simulink model "ass"  (Simulink 6.5)
settings: Solver=ode45  StartTime=0.0  StopTime=10.0  RelTol=1e-3
libraries: cdsFilt x333, cdsPhase x144, cdsRfmIO x26, cdsOsc x18, cdsMuxMatrix x8, cdsEpicsOut x3, cdsEzCaRead x1, cdsEpicsIn x1, cdsBitwise x1, cdsParameters x1
(part 3 of 17)

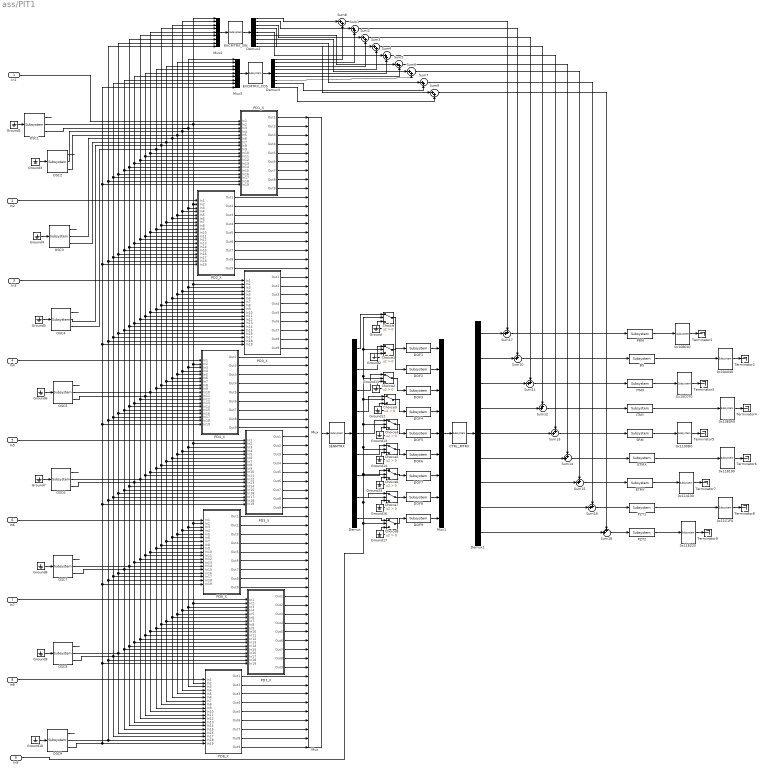
== system ass/PIT1 ==
  In1 : Inport
  In2 : Inport  Port=2
  In3 : Inport  Port=3
  In4 : Inport  Port=4
  In5 : Inport  Port=5
  In6 : Inport  Port=6
  In7 : Inport  Port=7
  In8 : Inport  Port=8
  In9 : Inport  Port=9
  0x108010 : cdsRfmIO/Subsystem  Tag=cdsRfmIO  Description=VMIC5565 Reflective Memory read/write  SystemSampleTime=-1
      settings: AttributesFormatString=%<Tag>
  0x10A040 : cdsRfmIO/Subsystem  Tag=cdsRfmIO  Description=VMIC5565 Reflective Memory read/write  SystemSampleTime=-1
      settings: AttributesFormatString=%<Tag>
  0x10C070 : cdsRfmIO/Subsystem  Tag=cdsRfmIO  Description=VMIC5565 Reflective Memory read/write  SystemSampleTime=-1
      settings: AttributesFormatString=%<Tag>
  0x10E0A0 : cdsRfmIO/Subsystem  Tag=cdsRfmIO  Description=VMIC5565 Reflective Memory read/write  SystemSampleTime=-1
      settings: AttributesFormatString=%<Tag>
  0x1100D0 : cdsRfmIO/Subsystem  Tag=cdsRfmIO  Description=VMIC5565 Reflective Memory read/write  SystemSampleTime=-1
      settings: AttributesFormatString=%<Tag>
  0x114130 : cdsRfmIO/Subsystem  Tag=cdsRfmIO  Description=VMIC5565 Reflective Memory read/write  SystemSampleTime=-1
      settings: AttributesFormatString=%<Tag>
  0x118190 : cdsRfmIO/Subsystem  Tag=cdsRfmIO  Description=VMIC5565 Reflective Memory read/write  SystemSampleTime=-1
      settings: AttributesFormatString=%<Tag>
  0x11C1F0 : cdsRfmIO/Subsystem  Tag=cdsRfmIO  Description=VMIC5565 Reflective Memory read/write  SystemSampleTime=-1
      settings: AttributesFormatString=%<Tag>
  0x11E220 : cdsRfmIO/Subsystem  Tag=cdsRfmIO  Description=VMIC5565 Reflective Memory read/write  SystemSampleTime=-1
      settings: AttributesFormatString=%<Tag>
  BS : cdsFilt/Subsystem  Tag=cdsFilt  Description=|  SystemSampleTime=-1
      | Purpose:                                                                                                                                                                                                                                  
      | Standard CDS IIR filter module.                                                                                                                                                                                                           
      |                                                                                                                                                                                                                                           
      | Operation:                                                                                                                                                                                                                                
      | Consists of 10 second order section IIR filters, plus a ramped gain stage. In FE code, also provides pre-defined test points and excitation channel inputs. The filter coefficients are defined in the LIGO system using the 'foton' tool.
      |                                                                                                                                                                                                                                           
      | Usage:                                                                                                                                                                                                                                    
      | Name the part with the desired filter module name.
      settings: AttributesFormatString=%<Tag>
  CTRL_MTRX : cdsMuxMatrix/Subsystem  Tag=cdsMuxMatrix  Description=Any size matrix. Inputs and outputs must be connected using Mux and Demux parts.  SystemSampleTime=-1
      settings: AttributesFormatString=%<Tag>
  Choice{,1..8} (9 alike) : Switch  Criteria=u2 > Threshold
  DOF1 : cdsFilt/Subsystem  Tag=cdsFilt  Description=|  SystemSampleTime=-1
      | Purpose:                                                                                                                                                                                                                                  
      | Standard CDS IIR filter module.                                                                                                                                                                                                           
      |                                                                                                                                                                                                                                           
      | Operation:                                                                                                                                                                                                                                
      | Consists of 10 second order section IIR filters, plus a ramped gain stage. In FE code, also provides pre-defined test points and excitation channel inputs. The filter coefficients are defined in the LIGO system using the 'foton' tool.
      |                                                                                                                                                                                                                                           
      | Usage:                                                                                                                                                                                                                                    
      | Name the part with the desired filter module name.
      settings: AttributesFormatString=%<Tag>
  DOF2 : cdsFilt/Subsystem  Tag=cdsFilt  Description=|  SystemSampleTime=-1
      | Purpose:                                                                                                                                                                                                                                  
      | Standard CDS IIR filter module.                                                                                                                                                                                                           
      |                                                                                                                                                                                                                                           
      | Operation:                                                                                                                                                                                                                                
      | Consists of 10 second order section IIR filters, plus a ramped gain stage. In FE code, also provides pre-defined test points and excitation channel inputs. The filter coefficients are defined in the LIGO system using the 'foton' tool.
      |                                                                                                                                                                                                                                           
      | Usage:                                                                                                                                                                                                                                    
      | Name the part with the desired filter module name.
      settings: AttributesFormatString=%<Tag>
  DOF3 : cdsFilt/Subsystem  Tag=cdsFilt  Description=|  SystemSampleTime=-1
      | Purpose:                                                                                                                                                                                                                                  
      | Standard CDS IIR filter module.                                                                                                                                                                                                           
      |                                                                                                                                                                                                                                           
      | Operation:                                                                                                                                                                                                                                
      | Consists of 10 second order section IIR filters, plus a ramped gain stage. In FE code, also provides pre-defined test points and excitation channel inputs. The filter coefficients are defined in the LIGO system using the 'foton' tool.
      |                                                                                                                                                                                                                                           
      | Usage:                                                                                                                                                                                                                                    
      | Name the part with the desired filter module name.
      settings: AttributesFormatString=%<Tag>
  DOF4 : cdsFilt/Subsystem  Tag=cdsFilt  Description=|  SystemSampleTime=-1
      | Purpose:                                                                                                                                                                                                                                  
      | Standard CDS IIR filter module.                                                                                                                                                                                                           
      |                                                                                                                                                                                                                                           
      | Operation:                                                                                                                                                                                                                                
      | Consists of 10 second order section IIR filters, plus a ramped gain stage. In FE code, also provides pre-defined test points and excitation channel inputs. The filter coefficients are defined in the LIGO system using the 'foton' tool.
      |                                                                                                                                                                                                                                           
      | Usage:                                                                                                                                                                                                                                    
      | Name the part with the desired filter module name.
      settings: AttributesFormatString=%<Tag>
  DOF5 : cdsFilt/Subsystem  Tag=cdsFilt  Description=|  SystemSampleTime=-1
      | Purpose:                                                                                                                                                                                                                                  
      | Standard CDS IIR filter module.                                                                                                                                                                                                           
      |                                                                                                                                                                                                                                           
      | Operation:                                                                                                                                                                                                                                
      | Consists of 10 second order section IIR filters, plus a ramped gain stage. In FE code, also provides pre-defined test points and excitation channel inputs. The filter coefficients are defined in the LIGO system using the 'foton' tool.
      |                                                                                                                                                                                                                                           
      | Usage:                                                                                                                                                                                                                                    
      | Name the part with the desired filter module name.
      settings: AttributesFormatString=%<Tag>
  DOF6 : cdsFilt/Subsystem  Tag=cdsFilt  Description=|  SystemSampleTime=-1
      | Purpose:                                                                                                                                                                                                                                  
      | Standard CDS IIR filter module.                                                                                                                                                                                                           
      |                                                                                                                                                                                                                                           
      | Operation:                                                                                                                                                                                                                                
      | Consists of 10 second order section IIR filters, plus a ramped gain stage. In FE code, also provides pre-defined test points and excitation channel inputs. The filter coefficients are defined in the LIGO system using the 'foton' tool.
      |                                                                                                                                                                                                                                           
      | Usage:                                                                                                                                                                                                                                    
      | Name the part with the desired filter module name.
      settings: AttributesFormatString=%<Tag>
  DOF7 : cdsFilt/Subsystem  Tag=cdsFilt  Description=|  SystemSampleTime=-1
      | Purpose:                                                                                                                                                                                                                                  
      | Standard CDS IIR filter module.                                                                                                                                                                                                           
      |                                                                                                                                                                                                                                           
      | Operation:                                                                                                                                                                                                                                
      | Consists of 10 second order section IIR filters, plus a ramped gain stage. In FE code, also provides pre-defined test points and excitation channel inputs. The filter coefficients are defined in the LIGO system using the 'foton' tool.
      |                                                                                                                                                                                                                                           
      | Usage:                                                                                                                                                                                                                                    
      | Name the part with the desired filter module name.
      settings: AttributesFormatString=%<Tag>
  DOF8 : cdsFilt/Subsystem  Tag=cdsFilt  Description=|  SystemSampleTime=-1
      | Purpose:                                                                                                                                                                                                                                  
      | Standard CDS IIR filter module.                                                                                                                                                                                                           
      |                                                                                                                                                                                                                                           
      | Operation:                                                                                                                                                                                                                                
      | Consists of 10 second order section IIR filters, plus a ramped gain stage. In FE code, also provides pre-defined test points and excitation channel inputs. The filter coefficients are defined in the LIGO system using the 'foton' tool.
      |                                                                                                                                                                                                                                           
      | Usage:                                                                                                                                                                                                                                    
      | Name the part with the desired filter module name.
      settings: AttributesFormatString=%<Tag>
  DOF9 : cdsFilt/Subsystem  Tag=cdsFilt  Description=|  SystemSampleTime=-1
      | Purpose:                                                                                                                                                                                                                                  
      | Standard CDS IIR filter module.                                                                                                                                                                                                           
      |                                                                                                                                                                                                                                           
      | Operation:                                                                                                                                                                                                                                
      | Consists of 10 second order section IIR filters, plus a ramped gain stage. In FE code, also provides pre-defined test points and excitation channel inputs. The filter coefficients are defined in the LIGO system using the 'foton' tool.
      |                                                                                                                                                                                                                                           
      | Usage:                                                                                                                                                                                                                                    
      | Name the part with the desired filter module name.
      settings: AttributesFormatString=%<Tag>
  Demux{,1..3} (4 alike) : Demux  Outputs=9
  ETMX : cdsFilt/Subsystem  Tag=cdsFilt  Description=|  SystemSampleTime=-1
      | Purpose:                                                                                                                                                                                                                                  
      | Standard CDS IIR filter module.                                                                                                                                                                                                           
      |                                                                                                                                                                                                                                           
      | Operation:                                                                                                                                                                                                                                
      | Consists of 10 second order section IIR filters, plus a ramped gain stage. In FE code, also provides pre-defined test points and excitation channel inputs. The filter coefficients are defined in the LIGO system using the 'foton' tool.
      |                                                                                                                                                                                                                                           
      | Usage:                                                                                                                                                                                                                                    
      | Name the part with the desired filter module name.
      settings: AttributesFormatString=%<Tag>
  ETMY : cdsFilt/Subsystem  Tag=cdsFilt  Description=|  SystemSampleTime=-1
      | Purpose:                                                                                                                                                                                                                                  
      | Standard CDS IIR filter module.                                                                                                                                                                                                           
      |                                                                                                                                                                                                                                           
      | Operation:                                                                                                                                                                                                                                
      | Consists of 10 second order section IIR filters, plus a ramped gain stage. In FE code, also provides pre-defined test points and excitation channel inputs. The filter coefficients are defined in the LIGO system using the 'foton' tool.
      |                                                                                                                                                                                                                                           
      | Usage:                                                                                                                                                                                                                                    
      | Name the part with the desired filter module name.
      settings: AttributesFormatString=%<Tag>
  EXCMTRX_COS : cdsMuxMatrix/Subsystem  Tag=cdsMuxMatrix  Description=Any size matrix. Inputs and outputs must be connected using Mux and Demux parts.  SystemSampleTime=-1
      settings: AttributesFormatString=%<Tag>
  EXCMTRX_SIN : cdsMuxMatrix/Subsystem  Tag=cdsMuxMatrix  Description=Any size matrix. Inputs and outputs must be connected using Mux and Demux parts.  SystemSampleTime=-1
      settings: AttributesFormatString=%<Tag>
  Ground{,1..17} (18 alike) : Ground
  ITMX : cdsFilt/Subsystem  Tag=cdsFilt  Description=|  SystemSampleTime=-1
      | Purpose:                                                                                                                                                                                                                                  
      | Standard CDS IIR filter module.                                                                                                                                                                                                           
      |                                                                                                                                                                                                                                           
      | Operation:                                                                                                                                                                                                                                
      | Consists of 10 second order section IIR filters, plus a ramped gain stage. In FE code, also provides pre-defined test points and excitation channel inputs. The filter coefficients are defined in the LIGO system using the 'foton' tool.
      |                                                                                                                                                                                                                                           
      | Usage:                                                                                                                                                                                                                                    
      | Name the part with the desired filter module name.
      settings: AttributesFormatString=%<Tag>
  ITMY : cdsFilt/Subsystem  Tag=cdsFilt  Description=|  SystemSampleTime=-1
      | Purpose:                                                                                                                                                                                                                                  
      | Standard CDS IIR filter module.                                                                                                                                                                                                           
      |                                                                                                                                                                                                                                           
      | Operation:                                                                                                                                                                                                                                
      | Consists of 10 second order section IIR filters, plus a ramped gain stage. In FE code, also provides pre-defined test points and excitation channel inputs. The filter coefficients are defined in the LIGO system using the 'foton' tool.
      |                                                                                                                                                                                                                                           
      | Usage:                                                                                                                                                                                                                                    
      | Name the part with the desired filter module name.
      settings: AttributesFormatString=%<Tag>
  Mux : Mux  Inputs=72
  Mux1 : Mux  Inputs=9
  Mux2 : Mux  Inputs=9
  Mux3 : Mux  Inputs=9
  OSC{1..9} (9 alike) : cdsOsc/Subsystem  Tag=cdsOsc  Description=Oscillator  SystemSampleTime=-1
      settings: AttributesFormatString=%<Tag>
  PD1_X : Subsystem
  PD2_X : Subsystem
  PD3_X : Subsystem
  PD4_X : Subsystem
  PD5_X : Subsystem
  PD6_X : Subsystem
  PD7_X : Subsystem
  PD8_X : Subsystem
  PRM : cdsFilt/Subsystem  Tag=cdsFilt  Description=|  SystemSampleTime=-1
      | Purpose:                                                                                                                                                                                                                                  
      | Standard CDS IIR filter module.                                                                                                                                                                                                           
      |                                                                                                                                                                                                                                           
      | Operation:                                                                                                                                                                                                                                
      | Consists of 10 second order section IIR filters, plus a ramped gain stage. In FE code, also provides pre-defined test points and excitation channel inputs. The filter coefficients are defined in the LIGO system using the 'foton' tool.
      |                                                                                                                                                                                                                                           
      | Usage:                                                                                                                                                                                                                                    
      | Name the part with the desired filter module name.
      settings: AttributesFormatString=%<Tag>
  PZT1 : cdsFilt/Subsystem  Tag=cdsFilt  Description=|  SystemSampleTime=-1
      | Purpose:                                                                                                                                                                                                                                  
      | Standard CDS IIR filter module.                                                                                                                                                                                                           
      |                                                                                                                                                                                                                                           
      | Operation:                                                                                                                                                                                                                                
      | Consists of 10 second order section IIR filters, plus a ramped gain stage. In FE code, also provides pre-defined test points and excitation channel inputs. The filter coefficients are defined in the LIGO system using the 'foton' tool.
      |                                                                                                                                                                                                                                           
      | Usage:                                                                                                                                                                                                                                    
      | Name the part with the desired filter module name.
      settings: AttributesFormatString=%<Tag>
  PZT2 : cdsFilt/Subsystem  Tag=cdsFilt  Description=|  SystemSampleTime=-1
      | Purpose:                                                                                                                                                                                                                                  
      | Standard CDS IIR filter module.                                                                                                                                                                                                           
      |                                                                                                                                                                                                                                           
      | Operation:                                                                                                                                                                                                                                
      | Consists of 10 second order section IIR filters, plus a ramped gain stage. In FE code, also provides pre-defined test points and excitation channel inputs. The filter coefficients are defined in the LIGO system using the 'foton' tool.
      |                                                                                                                                                                                                                                           
      | Usage:                                                                                                                                                                                                                                    
      | Name the part with the desired filter module name.
      settings: AttributesFormatString=%<Tag>
  SENMTRX : cdsMuxMatrix/Subsystem  Tag=cdsMuxMatrix  Description=Any size matrix. Inputs and outputs must be connected using Mux and Demux parts.  SystemSampleTime=-1
      settings: AttributesFormatString=%<Tag>
  SRM : cdsFilt/Subsystem  Tag=cdsFilt  Description=|  SystemSampleTime=-1
      | Purpose:                                                                                                                                                                                                                                  
      | Standard CDS IIR filter module.                                                                                                                                                                                                           
      |                                                                                                                                                                                                                                           
      | Operation:                                                                                                                                                                                                                                
      | Consists of 10 second order section IIR filters, plus a ramped gain stage. In FE code, also provides pre-defined test points and excitation channel inputs. The filter coefficients are defined in the LIGO system using the 'foton' tool.
      |                                                                                                                                                                                                                                           
      | Usage:                                                                                                                                                                                                                                    
      | Name the part with the desired filter module name.
      settings: AttributesFormatString=%<Tag>
  Sum{1..9} (9 alike) : Sum  Inputs=|++
  Sum{10..18} (9 alike) : Sum  Inputs=++|
  Terminator{1..9} (9 alike) : Terminator
  wires:
  Ground1/1 -> OSC1/1
  PD1_X/1(Out1) -> Mux/1
  Mux/1 -> SENMTRX/1
  Mux1/1 -> CTRL_MTRX/1
  CTRL_MTRX/1 -> Demux1/1
  DOF1/1 -> Mux1/1
  DOF2/1 -> Mux1/2
  DOF3/1 -> Mux1/3
  DOF4/1 -> Mux1/4
  DOF5/1 -> Mux1/5
  DOF6/1 -> Mux1/6
  DOF7/1 -> Mux1/7
  DOF8/1 -> Mux1/8
  DOF9/1 -> Mux1/9
  0x108010/1 -> Terminator1/1
  0x10A040/1 -> Terminator2/1
  0x10C070/1 -> Terminator3/1
  0x10E0A0/1 -> Terminator4/1
  0x1100D0/1 -> Terminator5/1
  0x118190/1 -> Terminator6/1
  0x114130/1 -> Terminator7/1
  0x11C1F0/1 -> Terminator8/1
  0x11E220/1 -> Terminator9/1
  Ground3/1 -> OSC2/1
  Ground4/1 -> OSC3/1
  Ground5/1 -> OSC4/1
  Ground6/1 -> OSC5/1
  Ground7/1 -> OSC6/1
  Ground8/1 -> OSC7/1
  Ground9/1 -> OSC8/1
  Ground10/1 -> OSC9/1
  PD1_X/2(Out2) -> Mux/2
  PD1_X/3(Out3) -> Mux/3
  PD1_X/4(Out4) -> Mux/4
  PD1_X/5(Out5) -> Mux/5
  PD1_X/6(Out6) -> Mux/6
  PD1_X/7(Out7) -> Mux/7
  PD1_X/8(Out8) -> Mux/8
  PD1_X/9(Out9) -> Mux/9
  PD2_X/1(Out1) -> Mux/10
  PD2_X/2(Out2) -> Mux/11
  PD2_X/3(Out3) -> Mux/12
  PD2_X/4(Out4) -> Mux/13
  PD2_X/5(Out5) -> Mux/14
  PD2_X/6(Out6) -> Mux/15
  PD2_X/7(Out7) -> Mux/16
  PD2_X/8(Out8) -> Mux/17
  PD2_X/9(Out9) -> Mux/18
  PD3_X/1(Out1) -> Mux/19
  PD3_X/2(Out2) -> Mux/20
  PD3_X/3(Out3) -> Mux/21
  PD3_X/4(Out4) -> Mux/22
  PD3_X/5(Out5) -> Mux/23
  PD3_X/6(Out6) -> Mux/24
  PD3_X/7(Out7) -> Mux/25
  PD3_X/8(Out8) -> Mux/26
  PD3_X/9(Out9) -> Mux/27
  PD4_X/1(Out1) -> Mux/28
  PD4_X/2(Out2) -> Mux/29
  PD4_X/3(Out3) -> Mux/30
  PD4_X/4(Out4) -> Mux/31
  PD4_X/5(Out5) -> Mux/32
  PD4_X/6(Out6) -> Mux/33
  PD4_X/7(Out7) -> Mux/34
  PD4_X/8(Out8) -> Mux/35
  PD4_X/9(Out9) -> Mux/36
  PD5_X/1(Out1) -> Mux/37
  PD5_X/2(Out2) -> Mux/38
  PD5_X/3(Out3) -> Mux/39
  PD5_X/4(Out4) -> Mux/40
  PD5_X/5(Out5) -> Mux/41
  PD5_X/6(Out6) -> Mux/42
  PD5_X/7(Out7) -> Mux/43
  PD5_X/8(Out8) -> Mux/44
  PD5_X/9(Out9) -> Mux/45
  PD6_X/1(Out1) -> Mux/46
  PD6_X/2(Out2) -> Mux/47
  PD6_X/3(Out3) -> Mux/48
  PD6_X/4(Out4) -> Mux/49
  PD6_X/5(Out5) -> Mux/50
  PD6_X/6(Out6) -> Mux/51
  PD6_X/7(Out7) -> Mux/52
  PD6_X/8(Out8) -> Mux/53
  PD6_X/9(Out9) -> Mux/54
  PD7_X/1(Out1) -> Mux/55
  PD7_X/2(Out2) -> Mux/56
  PD7_X/3(Out3) -> Mux/57
  PD7_X/4(Out4) -> Mux/58
  PD7_X/5(Out5) -> Mux/59
  PD7_X/6(Out6) -> Mux/60
  PD7_X/7(Out7) -> Mux/61
  PD7_X/8(Out8) -> Mux/62
  PD7_X/9(Out9) -> Mux/63
  PD8_X/1(Out1) -> Mux/64
  PD8_X/2(Out2) -> Mux/65
  PD8_X/3(Out3) -> Mux/66
  PD8_X/4(Out4) -> Mux/67
  PD8_X/5(Out5) -> Mux/68
  PD8_X/6(Out6) -> Mux/69
  PD8_X/7(Out7) -> Mux/70
  PD8_X/8(Out8) -> Mux/71
  PD8_X/9(Out9) -> Mux/72
  OSC1/2 -> PD1_X/2(In2), PD7_X/2(In2), PD8_X/2(In2), PD6_X/2(In2), PD5_X/2(In2), PD4_X/2(In2), PD3_X/2(In2), PD2_X/2(In2), Mux2/1
  Mux2/1 -> EXCMTRX_SIN/1
  EXCMTRX_SIN/1 -> Demux2/1
  Mux3/1 -> EXCMTRX_COS/1
  EXCMTRX_COS/1 -> Demux3/1
  OSC1/3 -> PD7_X/3(In3), PD8_X/3(In3), PD6_X/3(In3), PD5_X/3(In3), PD4_X/3(In3), PD3_X/3(In3), PD2_X/3(In3), PD1_X/3(In3), Mux3/1
  OSC2/2 -> PD1_X/4(In4), Mux2/2, PD7_X/4(In4), PD8_X/4(In4), PD6_X/4(In4), PD5_X/4(In4), PD4_X/4(In4), PD3_X/4(In4), PD2_X/4(In4)
  OSC2/3 -> PD1_X/5(In5), Mux3/2, PD7_X/5(In5), PD8_X/5(In5), PD6_X/5(In5), PD5_X/5(In5), PD4_X/5(In5), PD3_X/5(In5), PD2_X/5(In5)
  OSC3/2 -> PD1_X/6(In6), Mux2/3, PD7_X/6(In6), PD8_X/6(In6), PD6_X/6(In6), PD5_X/6(In6), PD4_X/6(In6), PD3_X/6(In6), PD2_X/6(In6)
  OSC3/3 -> PD1_X/7(In7), Mux3/3, PD7_X/7(In7), PD8_X/7(In7), PD6_X/7(In7), PD5_X/7(In7), PD4_X/7(In7), PD3_X/7(In7), PD2_X/7(In7)
  OSC4/2 -> PD1_X/8(In8), PD7_X/8(In8), PD8_X/8(In8), PD6_X/8(In8), PD5_X/8(In8), PD4_X/8(In8), PD3_X/8(In8), PD2_X/8(In8), Mux2/4
  OSC4/3 -> PD1_X/9(In9), Mux3/4, PD7_X/9(In9), PD8_X/9(In9), PD6_X/9(In9), PD5_X/9(In9), PD4_X/9(In9), PD3_X/9(In9), PD2_X/9(In9)
  OSC5/2 -> PD1_X/10(In10), Mux2/5, PD2_X/10(In10), PD3_X/10(In10), PD7_X/10(In10), PD8_X/10(In10), PD6_X/10(In10), PD5_X/10(In10), PD4_X/10(In10)
  OSC5/3 -> PD1_X/11(In11), Mux3/5, PD2_X/11(In11), PD3_X/11(In11), PD7_X/11(In11), PD8_X/11(In11), PD6_X/11(In11), PD5_X/11(In11), PD4_X/11(In11)
  OSC6/2 -> PD1_X/12(In12), Mux2/6, PD2_X/12(In12), PD3_X/12(In12), PD4_X/12(In12), PD7_X/12(In12), PD8_X/12(In12), PD6_X/12(In12), PD5_X/12(In12)
  OSC6/3 -> PD1_X/13(In13), Mux3/6, PD2_X/13(In13), PD3_X/13(In13), PD4_X/13(In13), PD7_X/13(In13), PD8_X/13(In13), PD6_X/13(In13), PD5_X/13(In13)
  OSC7/2 -> PD1_X/14(In14), Mux2/7, PD2_X/14(In14), PD3_X/14(In14), PD4_X/14(In14), PD5_X/14(In14), PD7_X/14(In14), PD8_X/14(In14), PD6_X/14(In14)
  OSC7/3 -> PD1_X/15(In15), Mux3/7, PD2_X/15(In15), PD3_X/15(In15), PD4_X/15(In15), PD5_X/15(In15), PD7_X/15(In15), PD8_X/15(In15), PD6_X/15(In15)
  OSC8/2 -> PD1_X/16(In16), Mux2/8, PD2_X/16(In16), PD3_X/16(In16), PD4_X/16(In16), PD5_X/16(In16), PD6_X/16(In16), PD7_X/16(In16), PD8_X/16(In16)
  OSC8/3 -> PD1_X/17(In17), Mux3/8, PD2_X/17(In17), PD3_X/17(In17), PD4_X/17(In17), PD5_X/17(In17), PD6_X/17(In17), PD7_X/17(In17), PD8_X/17(In17)
  OSC9/2 -> PD1_X/18(In18), Mux2/9, PD2_X/18(In18), PD3_X/18(In18), PD4_X/18(In18), PD5_X/18(In18), PD6_X/18(In18), PD7_X/18(In18), PD8_X/18(In18)
  OSC9/3 -> PD1_X/19(In19), Mux3/9, PD2_X/19(In19), PD3_X/19(In19), PD4_X/19(In19), PD5_X/19(In19), PD6_X/19(In19), PD7_X/19(In19), PD8_X/19(In19)
  Demux2/1 -> Sum8/1
  Demux3/1 -> Sum8/2
  Demux2/2 -> Sum1/1
  Demux3/2 -> Sum1/2
  Demux3/3 -> Sum2/2
  Demux2/3 -> Sum2/1
  Demux3/4 -> Sum3/2
  Demux2/4 -> Sum3/1
  Demux3/5 -> Sum4/2
  Demux3/6 -> Sum5/2
  Demux3/7 -> Sum6/2
  Demux3/9 -> Sum9/2
  Demux3/8 -> Sum7/2
  Demux2/5 -> Sum4/1
  Demux2/6 -> Sum5/1
  Demux2/7 -> Sum6/1
  Demux2/8 -> Sum7/1
  Demux2/9 -> Sum9/1
  Demux1/1 -> Sum17/2
  Demux1/2 -> Sum10/2
  Demux1/3 -> Sum11/2
  Sum8/1 -> Sum17/1
  Sum1/1 -> Sum10/1
  Sum2/1 -> Sum11/1
  Demux1/4 -> Sum12/2
  Sum3/1 -> Sum12/1
  Demux1/5 -> Sum13/2
  Sum4/1 -> Sum13/1
  Demux1/6 -> Sum14/2
  Sum5/1 -> Sum14/1
  Sum17/1 -> PRM/1
  Sum10/1 -> BS/1
  Sum11/1 -> ITMX/1
  Sum12/1 -> ITMY/1
  Sum13/1 -> SRM/1
  Sum14/1 -> ETMX/1
  Demux1/7 -> Sum15/2
  Sum15/1 -> ETMY/1
  Sum6/1 -> Sum15/1
  Demux1/8 -> Sum16/2
  Demux1/9 -> Sum18/2
  Sum18/1 -> PZT2/1
  Sum16/1 -> PZT1/1
  Sum7/1 -> Sum16/1
  Sum9/1 -> Sum18/1
  OSC1/1 -> ?
  In1/1 -> PD1_X/1(In1)
  OSC2/1 -> ?
  In2/1 -> PD2_X/1(In1)
  OSC3/1 -> ?
  In3/1 -> PD3_X/1(In1)
  OSC4/1 -> ?
  In4/1 -> PD4_X/1(In1)
  OSC5/1 -> ?
  In5/1 -> PD5_X/1(In1)
  OSC6/1 -> ?
  In6/1 -> PD6_X/1(In1)
  OSC7/1 -> ?
  In7/1 -> PD7_X/1(In1)
  OSC8/1 -> ?
  In8/1 -> PD8_X/1(In1)
  OSC9/1 -> ?
  PRM/1 -> 0x108010/1
  BS/1 -> 0x10A040/1
  ITMX/1 -> 0x10C070/1
  ITMY/1 -> 0x10E0A0/1
  SRM/1 -> 0x1100D0/1
  ETMX/1 -> 0x118190/1
  ETMY/1 -> 0x114130/1
  PZT1/1 -> 0x11C1F0/1
  PZT2/1 -> 0x11E220/1
  Ground/1 -> Choice/3
  In9/1 -> Choice/2, Choice1/2, Choice2/2, Choice3/2, Choice4/2, Choice5/2, Choice6/2, Choice7/2, Choice8/2
  SENMTRX/1 -> Demux/1
  Ground2/1 -> Choice1/3
  Demux/1 -> Choice/1
  Choice/1 -> DOF1/1
  Choice1/1 -> DOF2/1
  Demux/2 -> Choice1/1
  Ground11/1 -> Choice2/3
  Ground12/1 -> Choice3/3
  Ground13/1 -> Choice4/3
  Ground14/1 -> Choice5/3
  Ground15/1 -> Choice6/3
  Ground16/1 -> Choice7/3
  Demux/3 -> Choice2/1
  Choice2/1 -> DOF3/1
  Choice3/1 -> DOF4/1
  Demux/4 -> Choice3/1
  Choice4/1 -> DOF5/1
  Demux/5 -> Choice4/1
  Choice5/1 -> DOF6/1
  Demux/6 -> Choice5/1
  Choice6/1 -> DOF7/1
  Demux/7 -> Choice6/1
  Ground17/1 -> Choice8/3
  Choice7/1 -> DOF8/1
  Demux/8 -> Choice7/1
  Choice8/1 -> DOF9/1
  Demux/9 -> Choice8/1

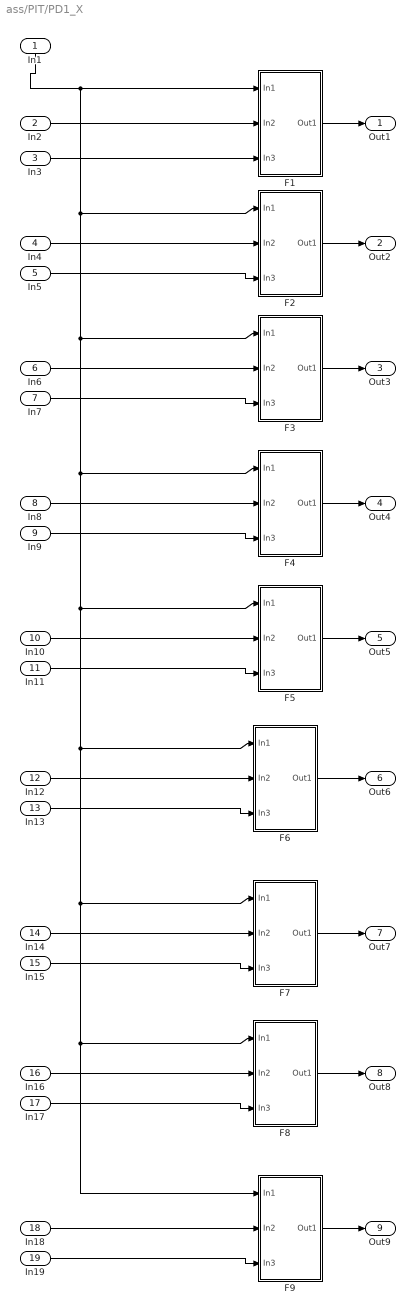
== system ass/PIT/PD1_X ==
  In1 : Inport  Orientation=down
  In2 : Inport  Port=2
  In3 : Inport  Port=3
  In4 : Inport  Port=4
  In5 : Inport  Port=5
  In6 : Inport  Port=6
  In7 : Inport  Port=7
  In8 : Inport  Port=8
  In9 : Inport  Port=9
  In10 : Inport  Port=10
  In11 : Inport  Port=11
  In12 : Inport  Port=12
  In13 : Inport  Port=13
  In14 : Inport  Port=14
  In15 : Inport  Port=15
  In16 : Inport  Port=16
  In17 : Inport  Port=17
  In18 : Inport  Port=18
  In19 : Inport  Port=19
  F1 : Subsystem
  F2 : Subsystem
  F3 : Subsystem
  F4 : Subsystem
  F5 : Subsystem
  F6 : Subsystem
  F7 : Subsystem
  F8 : Subsystem
  F9 : Subsystem
  Out1 : Outport
  Out2 : Outport  Port=2
  Out3 : Outport  Port=3
  Out4 : Outport  Port=4
  Out5 : Outport  Port=5
  Out6 : Outport  Port=6
  Out7 : Outport  Port=7
  Out8 : Outport  Port=8
  Out9 : Outport  Port=9
  wires:
  In1/1 -> F1/1(In1), F8/1(In1), F9/1(In1), F7/1(In1), F6/1(In1), F5/1(In1), F4/1(In1), F3/1(In1), F2/1(In1)
  In2/1 -> F1/2(In2)
  F1/1(Out1) -> Out1/1
  In3/1 -> F1/3(In3)
  In4/1 -> F2/2(In2)
  F2/1(Out1) -> Out2/1
  In5/1 -> F2/3(In3)
  In6/1 -> F3/2(In2)
  F3/1(Out1) -> Out3/1
  In7/1 -> F3/3(In3)
  In8/1 -> F4/2(In2)
  F4/1(Out1) -> Out4/1
  In9/1 -> F4/3(In3)
  In10/1 -> F5/2(In2)
  F5/1(Out1) -> Out5/1
  In11/1 -> F5/3(In3)
  In12/1 -> F6/2(In2)
  F6/1(Out1) -> Out6/1
  In13/1 -> F6/3(In3)
  In14/1 -> F7/2(In2)
  F7/1(Out1) -> Out7/1
  In15/1 -> F7/3(In3)
  In16/1 -> F8/2(In2)
  F8/1(Out1) -> Out8/1
  In17/1 -> F8/3(In3)
  In18/1 -> F9/2(In2)
  F9/1(Out1) -> Out9/1
  In19/1 -> F9/3(In3)

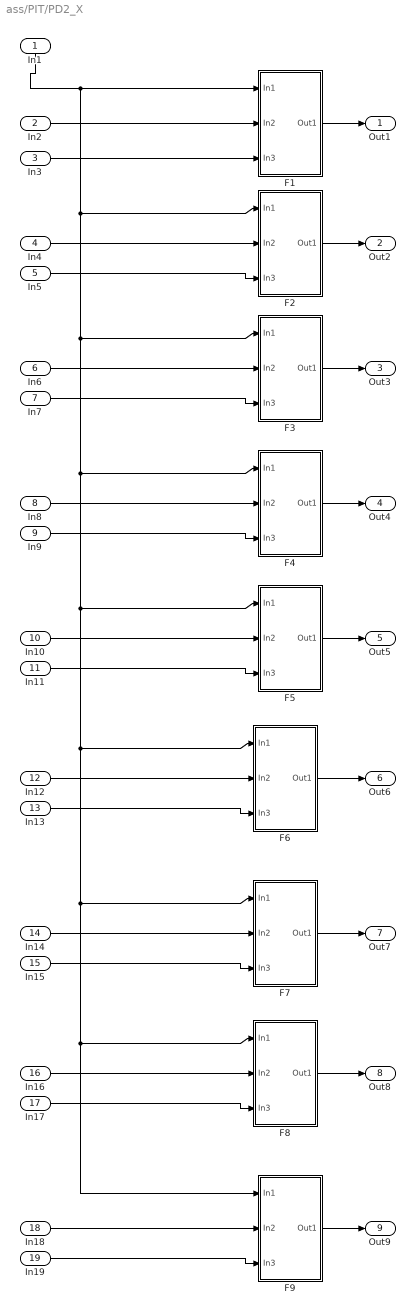
== system ass/PIT/PD2_X ==
  In1 : Inport  Orientation=down
  In2 : Inport  Port=2
  In3 : Inport  Port=3
  In4 : Inport  Port=4
  In5 : Inport  Port=5
  In6 : Inport  Port=6
  In7 : Inport  Port=7
  In8 : Inport  Port=8
  In9 : Inport  Port=9
  In10 : Inport  Port=10
  In11 : Inport  Port=11
  In12 : Inport  Port=12
  In13 : Inport  Port=13
  In14 : Inport  Port=14
  In15 : Inport  Port=15
  In16 : Inport  Port=16
  In17 : Inport  Port=17
  In18 : Inport  Port=18
  In19 : Inport  Port=19
  F1 : Subsystem
  F2 : Subsystem
  F3 : Subsystem
  F4 : Subsystem
  F5 : Subsystem
  F6 : Subsystem
  F7 : Subsystem
  F8 : Subsystem
  F9 : Subsystem
  Out1 : Outport
  Out2 : Outport  Port=2
  Out3 : Outport  Port=3
  Out4 : Outport  Port=4
  Out5 : Outport  Port=5
  Out6 : Outport  Port=6
  Out7 : Outport  Port=7
  Out8 : Outport  Port=8
  Out9 : Outport  Port=9
  wires:
  In1/1 -> F1/1(In1), F8/1(In1), F9/1(In1), F7/1(In1), F6/1(In1), F5/1(In1), F4/1(In1), F3/1(In1), F2/1(In1)
  In2/1 -> F1/2(In2)
  F1/1(Out1) -> Out1/1
  In3/1 -> F1/3(In3)
  In4/1 -> F2/2(In2)
  F2/1(Out1) -> Out2/1
  In5/1 -> F2/3(In3)
  In6/1 -> F3/2(In2)
  F3/1(Out1) -> Out3/1
  In7/1 -> F3/3(In3)
  In8/1 -> F4/2(In2)
  F4/1(Out1) -> Out4/1
  In9/1 -> F4/3(In3)
  In10/1 -> F5/2(In2)
  F5/1(Out1) -> Out5/1
  In11/1 -> F5/3(In3)
  In12/1 -> F6/2(In2)
  F6/1(Out1) -> Out6/1
  In13/1 -> F6/3(In3)
  In14/1 -> F7/2(In2)
  F7/1(Out1) -> Out7/1
  In15/1 -> F7/3(In3)
  In16/1 -> F8/2(In2)
  F8/1(Out1) -> Out8/1
  In17/1 -> F8/3(In3)
  In18/1 -> F9/2(In2)
  F9/1(Out1) -> Out9/1
  In19/1 -> F9/3(In3)

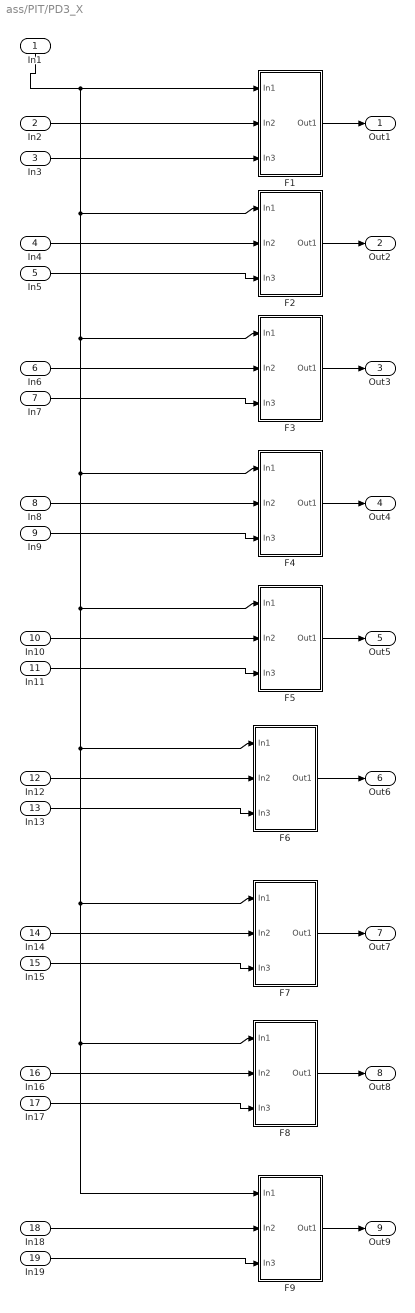
== system ass/PIT/PD3_X ==
  In1 : Inport  Orientation=down
  In2 : Inport  Port=2
  In3 : Inport  Port=3
  In4 : Inport  Port=4
  In5 : Inport  Port=5
  In6 : Inport  Port=6
  In7 : Inport  Port=7
  In8 : Inport  Port=8
  In9 : Inport  Port=9
  In10 : Inport  Port=10
  In11 : Inport  Port=11
  In12 : Inport  Port=12
  In13 : Inport  Port=13
  In14 : Inport  Port=14
  In15 : Inport  Port=15
  In16 : Inport  Port=16
  In17 : Inport  Port=17
  In18 : Inport  Port=18
  In19 : Inport  Port=19
  F1 : Subsystem
  F2 : Subsystem
  F3 : Subsystem
  F4 : Subsystem
  F5 : Subsystem
  F6 : Subsystem
  F7 : Subsystem
  F8 : Subsystem
  F9 : Subsystem
  Out1 : Outport
  Out2 : Outport  Port=2
  Out3 : Outport  Port=3
  Out4 : Outport  Port=4
  Out5 : Outport  Port=5
  Out6 : Outport  Port=6
  Out7 : Outport  Port=7
  Out8 : Outport  Port=8
  Out9 : Outport  Port=9
  wires:
  In1/1 -> F1/1(In1), F8/1(In1), F9/1(In1), F7/1(In1), F6/1(In1), F5/1(In1), F4/1(In1), F3/1(In1), F2/1(In1)
  In2/1 -> F1/2(In2)
  F1/1(Out1) -> Out1/1
  In3/1 -> F1/3(In3)
  In4/1 -> F2/2(In2)
  F2/1(Out1) -> Out2/1
  In5/1 -> F2/3(In3)
  In6/1 -> F3/2(In2)
  F3/1(Out1) -> Out3/1
  In7/1 -> F3/3(In3)
  In8/1 -> F4/2(In2)
  F4/1(Out1) -> Out4/1
  In9/1 -> F4/3(In3)
  In10/1 -> F5/2(In2)
  F5/1(Out1) -> Out5/1
  In11/1 -> F5/3(In3)
  In12/1 -> F6/2(In2)
  F6/1(Out1) -> Out6/1
  In13/1 -> F6/3(In3)
  In14/1 -> F7/2(In2)
  F7/1(Out1) -> Out7/1
  In15/1 -> F7/3(In3)
  In16/1 -> F8/2(In2)
  F8/1(Out1) -> Out8/1
  In17/1 -> F8/3(In3)
  In18/1 -> F9/2(In2)
  F9/1(Out1) -> Out9/1
  In19/1 -> F9/3(In3)
